simulink model "BFSKandPCM"  (R2018b)
settings: Solver=VariableStepAuto  StartTime=0.0  StopTime=160  RelTol=1e-3
libraries: dsparch4 x9, commsrccod2 x4, commutil2 x4, commsink2 x3, commchan3 x1
settings Model: Creator=lance  LastModifiedBy=lance

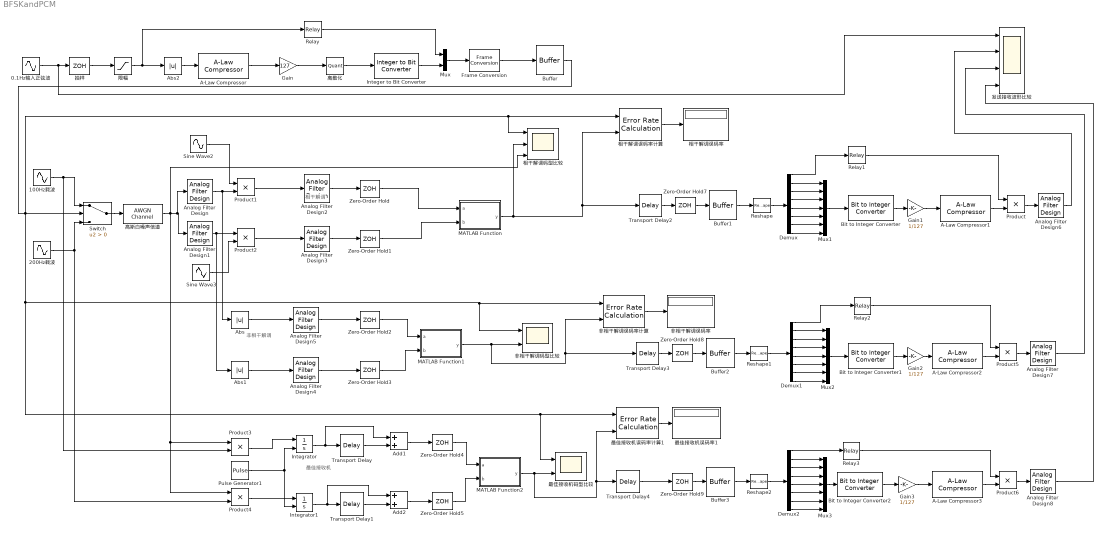
== system BFSKandPCM ==
  note: 非相干解调
  note: 相干解调
  note: 最佳接收机
  0.1Hz输入正弦波 : Sin  Frequency=0.1*2*pi  SampleTime=0.0001
  100Hz载波 : Sin  Frequency=100*2*pi  SampleTime=0.0001
  200Hz载波 : Sin  Frequency=200*2*pi  SampleTime=0.0001
  A-Law Compressor{,1..3} (4 alike) : commsrccod2/A-Law Compressor  A=87.6  V=1
      settings: SourceProductName=Communications System Toolbox  SourceProductBaseCode=CM
  Abs : Abs
  Abs1 : Abs
  Abs2 : Abs
  Add1 : Sum
  Add2 : Sum
  Analog Filter Design : dsparch4/Analog Filter Design  method=Butterworth  filttype=Bandpass  N=8  Wlo=90*2*pi  Whi=110*2*pi  Rp=2  Rs=40
  Analog Filter Design1 : dsparch4/Analog Filter Design  method=Butterworth  filttype=Bandpass  N=8  Wlo=190*2*pi  Whi=210*2*pi  Rp=2  Rs=40
  Analog Filter Design{2..5} (4 alike) : dsparch4/Analog Filter Design  method=Butterworth  filttype=Lowpass  N=8  Wlo=10*pi  Whi=103*2*pi  Rp=2  Rs=40
  Analog Filter Design6 : dsparch4/Analog Filter Design  method=Butterworth  filttype=Lowpass  N=8  Wlo=2*pi*0.2  Whi=210*2*pi  Rp=2  Rs=40
  Analog Filter Design7 : dsparch4/Analog Filter Design  method=Butterworth  filttype=Lowpass  N=8  Wlo=0.2*2*pi  Whi=210*2*pi  Rp=2  Rs=40
  Analog Filter Design8 : dsparch4/Analog Filter Design  method=Butterworth  filttype=Lowpass  N=8  Wlo=0.2*2*pi  Whi=210*2*pi  Rp=2  Rs=40
  Bit to Integer Converter : commutil2/Bit to Integer Converter  nbits=7  bitOrder=MSB first  signedOutputValues=Unsigned  outDtype=Inherit via internal rule  outDtypeSigned=Inherit via internal rule
  Bit to Integer Converter1 : commutil2/Bit to Integer Converter  nbits=7  bitOrder=MSB first  signedOutputValues=Unsigned  outDtype=Inherit via internal rule  outDtypeSigned=Inherit via internal rule
  Bit to Integer Converter2 : commutil2/Bit to Integer Converter  nbits=7  bitOrder=MSB first  signedOutputValues=Unsigned  outDtype=Inherit via internal rule  outDtypeSigned=Inherit via internal rule
  Buffer : Buffer  N=1  OutputFrames=off
  Buffer1 : Buffer  N=8  OutputFrames=off
  Buffer2 : Buffer  N=8  OutputFrames=off
  Buffer3 : Buffer  N=8  OutputFrames=off
  Demux : Demux  Outputs=8
  Demux1 : Demux  Outputs=8
  Demux2 : Demux  Outputs=8
  Frame Conversion : FrameConversion
  Gain : Gain  Gain=127
  Gain1 : Gain  Gain=1/127  SampleTime=0.2
  Gain2 : Gain  Gain=1/127  SampleTime=0.2
  Gain3 : Gain  Gain=1/127  SampleTime=0.2
  Integer to Bit Converter : commutil2/Integer to Bit Converter  nbits=7  signedInputValues=Unsigned  bitOrder=MSB first  outDtype=Inherit via internal rule
  Integrator : Integrator  ExternalReset=rising
  Integrator1 : Integrator  ExternalReset=rising
  MATLAB Function : MATLAB Function  TreatAsAtomicUnit=on
  MATLAB Function1 : MATLAB Function  TreatAsAtomicUnit=on
  MATLAB Function2 : MATLAB Function  TreatAsAtomicUnit=on
  Mux : Mux  Inputs=2
  Mux1 : Mux  Inputs=7
  Mux2 : Mux  Inputs=7
  Mux3 : Mux  Inputs=7
  Product : Product  RndMeth=Zero
  Product{1..4} (4 alike) : Product
  Product5 : Product  RndMeth=Zero
  Product6 : Product  RndMeth=Zero
  Pulse Generator1 : DiscretePulseGenerator  PulseType=Time based  Period=0.2
  Relay : Relay
  Relay1 : Relay  OffOutputValue=-1  SampleTime=0.001
  Relay2 : Relay  OffOutputValue=-1  SampleTime=0.001
  Relay3 : Relay  OffOutputValue=-1  SampleTime=0.001
  Reshape : Reshape
  Reshape1 : Reshape
  Reshape2 : Reshape
  Sine Wave2 : Sin  Frequency=100*2*pi  SampleTime=0.0001
  Sine Wave3 : Sin  Frequency=200*2*pi  SampleTime=0.0001
  Switch : Switch  Criteria=u2 > Threshold
  Transport Delay : TransportDelay  DelayTime=0.02
  Transport Delay1 : TransportDelay  DelayTime=0.02
  Transport Delay2 : TransportDelay  DelayTime=1.2
  Transport Delay3 : TransportDelay  DelayTime=1.2
  Transport Delay4 : TransportDelay  DelayTime=1.4
  Zero-Order Hold{,1..5,7..9} (9 alike) : ZeroOrderHold  SampleTime=0.2
  发送接收波形比较 : Scope  NumInputPorts=4
  抽样 : ZeroOrderHold  SampleTime=1.6
  最佳接收机码型比较 : Scope  NumInputPorts=2
  最佳接收机误码率1 : Display
  最佳接收机误码率计算1 : commsink2/Error Rate Calculation  N=1  st_delay=0  cp_mode=Entire frame  subframe=[]  PMode=Port  WsName=ErrorVec  RsMode2=off  stop=off  numErr=100  maxBits=1e6
  相干解调码型比较 : Scope  NumInputPorts=3
  相干解调误码率 : Display
  "相干解调误码率计算 " : commsink2/Error Rate Calculation  N=2  st_delay=0  cp_mode=Entire frame  subframe=[]  PMode=Port  WsName=ErrorVec  RsMode2=off  stop=off  numErr=100  maxBits=1e6
  离散化 : Quantizer  QuantizationInterval=1
  限幅 : Saturate  UpperLimit=1  LowerLimit=-1
  非相干解调码型比较 : Scope  NumInputPorts=2
  非相干解调误码率 : Display
  非相干解调误码率计算 : commsink2/Error Rate Calculation  N=2  st_delay=0  cp_mode=Entire frame  subframe=[]  PMode=Port  WsName=ErrorVec  RsMode2=off  stop=off  numErr=100  maxBits=1e6
  "高斯白噪声信道 " : commchan3/AWGN Channel  InputProcessing=Columns as channels (frame based)  seed=67  noiseMode="Signal to noise ratio  (SNR)"  EbNodB=1  EsNodB=10  SNRdB=-19  bitsPerSym=1  Ps=1  Tsym=1  variance=1
  wires:
  100Hz载波/1 -> Product3/2, Switch/1
  200Hz载波/1 -> Switch/3, Product4/2
  Sine Wave2/1 -> Product1/1
  Analog Filter Design/1 -> Abs/1, Product1/2
  Sine Wave3/1 -> Product2/2
  Analog Filter Design1/1 -> Abs1/1, Product2/1
  Product1/1 -> Analog Filter Design2/1
  Product2/1 -> Analog Filter Design3/1
  Analog Filter Design3/1 -> Zero-Order Hold1/1
  Analog Filter Design2/1 -> Zero-Order Hold/1
  "相干解调误码率计算 "/1 -> 相干解调误码率/1
  Zero-Order Hold/1 -> MATLAB Function/1(a)
  Zero-Order Hold1/1 -> MATLAB Function/2(b)
  MATLAB Function/1(y) -> 相干解调码型比较/2, "相干解调误码率计算 "/2, Transport Delay2/1
  Switch/1 -> "高斯白噪声信道 "/1
  "高斯白噪声信道 "/1 -> Product4/1, Product3/1, Analog Filter Design1/1, Analog Filter Design/1, 相干解调码型比较/3
  Abs/1 -> Analog Filter Design5/1
  Abs1/1 -> Analog Filter Design4/1
  Analog Filter Design5/1 -> Zero-Order Hold2/1
  Analog Filter Design4/1 -> Zero-Order Hold3/1
  Zero-Order Hold2/1 -> MATLAB Function1/1(a)
  Zero-Order Hold3/1 -> MATLAB Function1/2(b)
  非相干解调误码率计算/1 -> 非相干解调误码率/1
  Product3/1 -> Integrator/1
  Pulse Generator1/1 -> Integrator1/2, Integrator/2
  Product4/1 -> Integrator1/1
  Integrator1/1 -> Add2/1, Transport Delay1/1
  Integrator/1 -> Add1/1, Transport Delay/1
  Transport Delay/1 -> Add1/2
  Transport Delay1/1 -> Add2/2
  Zero-Order Hold4/1 -> MATLAB Function2/1(a)
  Zero-Order Hold5/1 -> MATLAB Function2/2(b)
  Add1/1 -> Zero-Order Hold4/1
  Add2/1 -> Zero-Order Hold5/1
  最佳接收机误码率计算1/1 -> 最佳接收机误码率1/1
  Buffer/1 -> 最佳接收机码型比较/1, 最佳接收机误码率计算1/1, 非相干解调误码率计算/1, 非相干解调码型比较/1, Switch/2, "相干解调误码率计算 "/1, 相干解调码型比较/1
  Gain/1 -> 离散化/1
  Integer to Bit Converter/1 -> Mux/2
  A-Law Compressor/1 -> Gain/1
  Mux/1 -> Frame Conversion/1
  Relay/1 -> Mux/1
  离散化/1 -> Integer to Bit Converter/1
  限幅/1 -> Relay/1, Abs2/1
  0.1Hz输入正弦波/1 -> 发送接收波形比较/1, 抽样/1
  Abs2/1 -> A-Law Compressor/1
  Frame Conversion/1 -> Buffer/1
  Transport Delay2/1 -> Zero-Order Hold7/1
  Zero-Order Hold7/1 -> Buffer1/1
  Buffer1/1 -> Reshape/1
  Demux/7 -> Mux1/6
  Demux/8 -> Mux1/7
  Demux/3 -> Mux1/2
  Demux/5 -> Mux1/4
  Demux/6 -> Mux1/5
  Demux/2 -> Mux1/1
  A-Law Compressor1/1 -> Product/2
  Demux/1 -> Relay1/1
  Reshape/1 -> Demux/1
  Demux/4 -> Mux1/3
  Bit to Integer Converter/1 -> Gain1/1
  Relay1/1 -> Product/1
  Gain1/1 -> A-Law Compressor1/1
  Mux1/1 -> Bit to Integer Converter/1
  抽样/1 -> 限幅/1
  MATLAB Function1/1(y) -> 非相干解调码型比较/2, Transport Delay3/1, 非相干解调误码率计算/2
  Mux2/1 -> Bit to Integer Converter1/1
  Demux1/1 -> Relay2/1
  Gain2/1 -> A-Law Compressor2/1
  Relay2/1 -> Product5/1
  Demux1/4 -> Mux2/3
  Bit to Integer Converter1/1 -> Gain2/1
  Demux1/5 -> Mux2/4
  Demux1/7 -> Mux2/6
  Transport Delay3/1 -> Zero-Order Hold8/1
  Demux1/2 -> Mux2/1
  Buffer2/1 -> Reshape1/1
  Zero-Order Hold8/1 -> Buffer2/1
  Demux1/6 -> Mux2/5
  Demux1/3 -> Mux2/2
  A-Law Compressor2/1 -> Product5/2
  Reshape1/1 -> Demux1/1
  Demux1/8 -> Mux2/7
  Mux3/1 -> Bit to Integer Converter2/1
  Demux2/1 -> Relay3/1
  Gain3/1 -> A-Law Compressor3/1
  Relay3/1 -> Product6/1
  Demux2/4 -> Mux3/3
  Bit to Integer Converter2/1 -> Gain3/1
  Demux2/5 -> Mux3/4
  Demux2/7 -> Mux3/6
  MATLAB Function2/1(y) -> Transport Delay4/1, 最佳接收机误码率计算1/2, 最佳接收机码型比较/2
  Demux2/2 -> Mux3/1
  Buffer3/1 -> Reshape2/1
  Zero-Order Hold9/1 -> Buffer3/1
  Demux2/6 -> Mux3/5
  Demux2/3 -> Mux3/2
  A-Law Compressor3/1 -> Product6/2
  Reshape2/1 -> Demux2/1
  Demux2/8 -> Mux3/7
  Product5/1 -> Analog Filter Design7/1
  Product6/1 -> Analog Filter Design8/1
  Product/1 -> Analog Filter Design6/1
  Transport Delay4/1 -> Zero-Order Hold9/1
  Analog Filter Design8/1 -> 发送接收波形比较/4
  Analog Filter Design7/1 -> 发送接收波形比较/3
  Analog Filter Design6/1 -> 发送接收波形比较/2

== matlab function BFSKandPCM/MATLAB Function1 ==
  data: a input; y output; b input
function y = fcn(a, b)
if(a>b)
    y=1;
else
    y=0;
end

== matlab function BFSKandPCM/MATLAB Function ==
  data: a input; y output; b input
function y = fcn(a, b)
if(a>b)
    y=1;
else
    y=0;
end

== matlab function BFSKandPCM/MATLAB Function2 ==
  data: a input; y output; b input
function y = fcn(a, b)
if(a>b)
    y=1;
else
    y=0;
end
